simulink model "DC_motor_pid_model"  (R2025a)
settings: Solver=VariableStepAuto  StartTime=0.0  StopTime=10.0  RelTol=1e-3
settings Model: Creator=sabreen  LastModifiedBy=sabreen

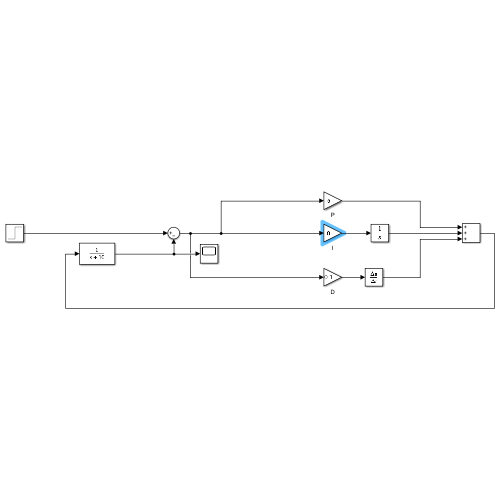
[thumbnail: Simulink's stored preview of the top-level diagram]
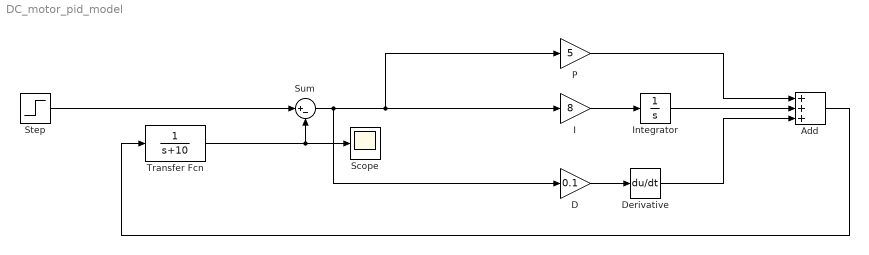
== system DC_motor_pid_model ==
  Add : Sum  Inputs=+++
  D : Gain  Gain=0.1
  Derivative : Derivative  CoefficientInTFapproximation=0.1
  I : Gain  Gain=8
  Integrator : Integrator
  P : Gain  Gain=5
  Scope : Scope
      settings: ActiveDisplayYMinimum=5.0148025288534894  ActiveDisplayYMaximum=10.894860707768572
  Step : Step  Time=0  After=10  SampleTime=0
  Sum : Sum  Inputs=|+-
  Transfer Fcn : TransferFcn  Denominator=[1 10]
  wires:
  Transfer Fcn/1 -> Scope/1, Sum/2
  Step/1 -> Sum/1
  Sum/1 -> I/1, P/1, D/1
  I/1 -> Integrator/1
  D/1 -> Derivative/1
  P/1 -> Add/1
  Integrator/1 -> Add/2
  Derivative/1 -> Add/3
  Add/1 -> Transfer Fcn/1
